simulink model "BT_Modell_WS1718"  (Simulink 8.6)
settings: Solver=FixedStepAuto  StartTime=0.0  StopTime=10  FixedStep=0.01  RelTol=1e-3
values from neighbouring files (symbols this model uses):
  c1 = 120*1000    (= 120000)    [BT_mfile_WS1718.m]
  c2 = 20*1000    (= 20000)    [BT_mfile_WS1718.m]
  cp = 0.5*1000    (= 500)    [BT_mfile_WS1718.m]
  d2 = 0.1*1000    (= 100)    [BT_mfile_WS1718.m]
  dp = 0.5*1000    (= 500)    [BT_mfile_WS1718.m]
  m1 = 30    [BT_mfile_WS1718.m]
  m2 = 250    [BT_mfile_WS1718.m]
  zh = 0.1    [BT_mfile_WS1718.m]
undefined symbols (not defined in the file or in its folder): sigbuilder_block
libraries: simulink x1
settings Model: Creator=wang  LastModifiedBy=wang
settings DataIOCC: SaveFormat=Dataset  SignalLoggingSaveFormat=Dataset
settings OptimizationCC: ExpressionDepthLimit=128
settings DebuggingCC: UnderspecifiedInitializationDetection=Simplified  MergeDetectMultiDrivingBlocksExec=error  SolverPrmCheckMsg=none  FcnCallInpInsideContextMsg=EnableAllAsError  StateNameClashWarn=none
settings HardwareCC: ProdBitPerPointer=64  ProdLargestAtomicFloat=Float  ProdIntDivRoundTo=Zero  ProdEndianess=LittleEndian  ProdWordSize=64  ProdHWDeviceType=Intel->x86-64 (Windows64)
settings GRTTargetCC: GeneratePreprocessorConditionals=Use local settings  CombineOutputUpdateFcns=on  GRTInterface=off
settings ConfigComp: CovModelRefEnable=off

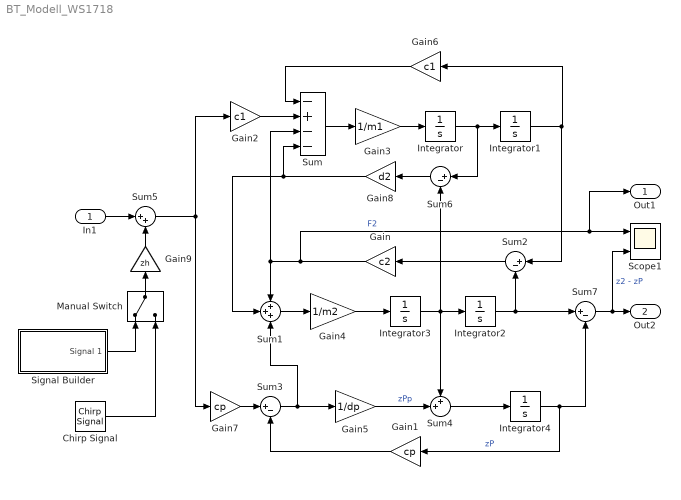
== system BT_Modell_WS1718 ==
  In1 : Inport
  Chirp Signal : simulink/Sources/Chirp Signal  f1=0.01  T=20  f2=20
  Gain : Gain  Gain=c2
  Gain1 : Gain  Gain=cp
  Gain2 : Gain  Gain=c1
  Gain3 : Gain  Gain=1/m1
  Gain4 : Gain  Gain=1/m2
  Gain5 : Gain  Gain=1/dp
  Gain6 : Gain  Gain=c1
  Gain7 : Gain  Gain=cp
  Gain8 : Gain  Gain=d2
  Gain9 : Gain  Gain=zh
  Integrator{,1..4} (5 alike) : Integrator
  Manual Switch : ManualSwitch
  Scope1 : Scope  NumInputPorts=2
  Signal Builder : Subsystem  Tag=STV Subsys  LoadFcn=sigbuilder_block('load');  StartFcn=sigbuilder_block('start');  StopFcn=sigbuilder_block('stop');  ClipboardFcn=sigbuilder_block('clipboard');  mask(Sigbuilder block){}
      mask help: Simulink:masks:SigbuilderBlock_MD
      mask init:
      | if ~strcmp(get_param(bdroot(gcbh),'SimulationStatus'),'stopped') tuvar = sigbuilder_block('maskInit'); end
      settings: CopyFcn=sigbuilder_block('copy');  DeleteFcn=sigbuilder_block('delete');  ModelCloseFcn=sigbuilder_block('modelClose');  PreSaveFcn=sigbuilder_block('preSave');  PauseFcn=sigbuilder_block('pause');  ContinueFcn=sigbuilder_block('continue');  NameChangeFcn=sigbuilder_block('namechange');  OpenFcn=sigbuilder_block('open',[51.5 84 550.5 362.5 ]);  CloseFcn=sigbuilder_block('close');
      mask Display: plot(0, 0, 100, 100,[2, 2, 32, 32, 2], [68, 8, 8, 68, 68],[32, 2], [38, 38], [32, 19, 2],[53, 60, 44], [32, 17, 17, 2],[16, 16, 31, 31]);txt = getActiveGroup(gcbh);text(2, 100, txt,'verticalAlignment', 'top');
  Sum : Sum  Inputs=-+--
  Sum1 : Sum  Inputs=+++
  Sum{2..3,6..7} (4 alike) : Sum  Inputs=|+-
  Sum4 : Sum  Inputs=++|
  Sum5 : Sum  Inputs=|++
  Out1 : Outport
  Out2 : Outport  Port=2
  wires:
  Sum/1 -> Gain3/1
  Gain2/1 -> Sum/2
  Gain3/1 -> Integrator/1
  Integrator/1 -> Sum6/1, Integrator1/1
  Sum1/1 -> Gain4/1
  Integrator1/1 -> Sum2/1, Gain6/1
  Gain6/1 -> Sum/1
  Sum2/1 -> Gain/1
  Gain7/1 -> Sum3/1
  Sum3/1 -> Gain5/1, Sum1/3
  Gain4/1 -> Integrator3/1
  Integrator3/1 -> Sum4/1, Sum6/2, Integrator2/1
  Integrator2/1 -> Sum7/1, Sum2/2
  Integrator4/1 -> Sum7/2, Gain1/1  "zP"
  Gain1/1 -> Sum3/2
  In1/1 -> Sum5/1
  Signal Builder/1(Signal 1) -> Manual Switch/1
  Sum5/1 -> Gain7/1, Gain2/1
  Manual Switch/1 -> Gain9/1
  Chirp Signal/1 -> Manual Switch/2
  Sum6/1 -> Gain8/1
  Gain8/1 -> Sum1/2, Sum/4
  Gain/1 -> Out1/1, Scope1/1, Sum/3, Sum1/1  "F2"
  Sum4/1 -> Integrator4/1
  Gain5/1 -> Sum4/2  "zPp"
  Sum7/1 -> Scope1/2, Out2/1  "z2 - zP"
  Gain9/1 -> Sum5/2

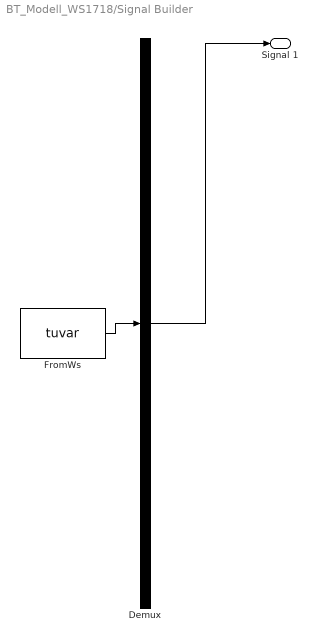
== system BT_Modell_WS1718/Signal Builder ==
  Demux : Demux  Tag=STV Demux  Outputs=1
  FromWs : FromWorkspace  Tag=STV FromWs  VariableName=tuvar  SampleTime=0  SigBuilderData=DataTag0  VnvData=DataTag1
      SigBuilderData=|
      | common.afterFinalStr = 'Extrapolate'
      | common.sampleTime = 0
      | dataSet.timeRange = [0 10]
      | dataSet.name = 'Group 1'
      | sbobj.Groups.Name = 'Group 1'
      | sbobj.Groups.Signals.Name = 'Signal 1'
      | sbobj.Groups.Signals.XData = [0 0.25 1.9 2 10]
      | sbobj.Groups.Signals.YData = [0 1 1 0 0]
  Signal 1 : Outport  Tag=STV Outport
  wires:
  Demux/1 -> Signal 1/1
  FromWs/1 -> Demux/1
